simulink model "model_new"  (R2016b)
settings: Solver=FixedStepAuto  StartTime=0.0  StopTime=10.0  RelTol=1e-3
undefined symbols (not defined in the file): magnitude
settings Model: Creator=202008840  LastModifiedBy=202008840
settings OptimizationCC: DefaultParameterBehavior=Inlined  UseDivisionForNetSlopeComputation=on  UseFloatMulNetSlope=on  InlineInvariantSignals=on  PassReuseOutputArgsAs=Individual arguments  ZeroExternalMemoryAtStartup=off  ZeroInternalMemoryAtStartup=off  NoFixptDivByZeroProtection=on  EfficientFloat2IntCast=on  LifeSpan=1
settings DebuggingCC: ParameterTunabilityLossMsg=error
settings RTWCC: SystemTargetFile=ert.tlc  TemplateMakefile=ert_default_tmf  Description=Embedded Coder  GenerateReport=on  IncludeHyperlinkInReport=on  LaunchReport=on  GenerateTraceInfo=on  GenerateTraceReport=on  GenerateTraceReportSl=on  GenerateTraceReportSf=on  GenerateTraceReportEml=on  GenerateCodeMetricsReport=on
settings CodeAppCC: ForceParamTrailComments=on  IgnoreCustomStorageClasses=off  OperatorAnnotations=on  SimulinkDataObjDesc=on  SFDataObjDesc=on  MATLABFcnDesc=on  CustomSymbolStrGlobalVar=rt$N$M  CustomSymbolStrType=$N$M  CustomSymbolStrFcn=$N$M$F  CustomSymbolStrMacro=$N$M  InsertBlockDesc=on  MATLABSourceComments=on
settings ERTTargetCC: TargetLangStandard=C99 (ISO)  GenerateSampleERTMain=on  CombineSignalStateStructs=on  SupportAbsoluteTime=off  SupportComplex=off  SupportContinuousTime=on  InlinedParameterPlacement=NonHierarchical  ERTCustomFileTemplate=example_file_process.tlc  ERTFilePackagingFormat=CompactWithDataFile

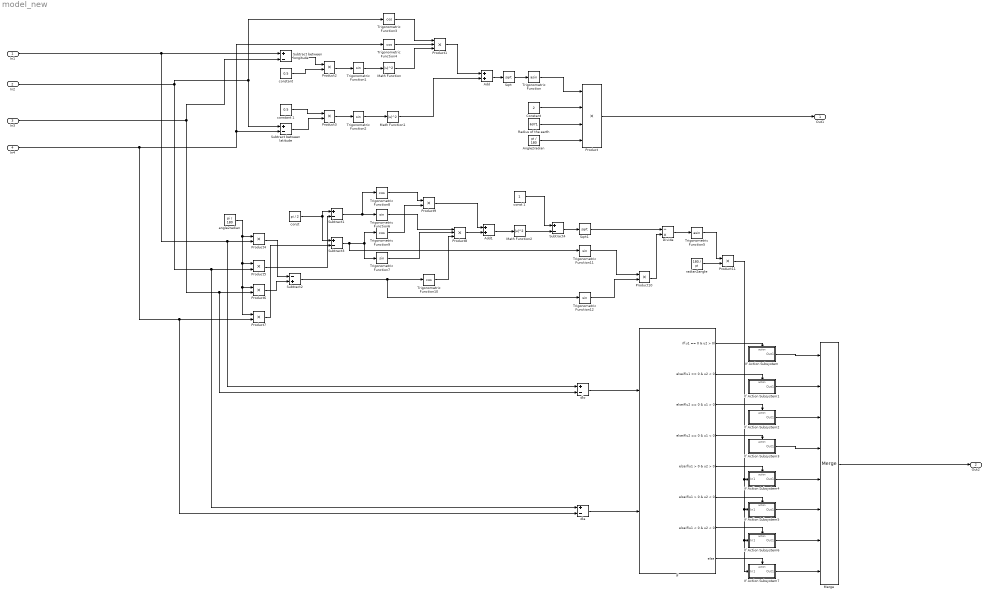
== system model_new ==
  In1 : Inport
  In2 : Inport  Port=2
  In3 : Inport  Port=3
  In4 : Inport  Port=4
  Add : Sum
  Add1 : Sum
  Angle2radian : Constant  Value=pi / 180
  Constant : Constant  Value=2
  Divide : Product  Inputs=/*
  If : If  NumInputs=2  IfExpression=u1 == 0 & u2 > 0  ElseIfExpressions=u1 == 0 & u2 < 0, u2 == 0 & u1 > 0, u2 == 0 & u1 < 0, u1 > 0 & u2 > 0, u1 > 0 & u2 < 0, u1 < 0 & u2 < 0
  If Action Subsystem : Subsystem  TreatAsAtomicUnit=on
  If Action Subsystem1 : Subsystem  TreatAsAtomicUnit=on
  If Action Subsystem2 : Subsystem  TreatAsAtomicUnit=on
  If Action Subsystem3 : Subsystem  TreatAsAtomicUnit=on
  If Action Subsystem4 : Subsystem  TreatAsAtomicUnit=on
  If Action Subsystem5 : Subsystem  TreatAsAtomicUnit=on
  If Action Subsystem6 : Subsystem  TreatAsAtomicUnit=on
  If Action Subsystem7 : Subsystem  TreatAsAtomicUnit=on
  Math Function : Math  Operator=magnitude^2  SaturateOnIntegerOverflow=on
  Math Function1 : Math  Operator=magnitude^2  SaturateOnIntegerOverflow=on
  Math Function2 : Math  Operator=magnitude^2  SaturateOnIntegerOverflow=on
  Merge : Merge  Inputs=8
  Product : Product  Inputs=4
  Product1 : Product  Inputs=3
  Product{2..7,9..11} (9 alike) : Product
  Product8 : Product  Inputs=3
  Radius of the earth : Constant  Value=6371
  Sqrt : Sqrt  SaturateOnIntegerOverflow=on
  Sqrt1 : Sqrt  SaturateOnIntegerOverflow=on
  Subtract between latitude : Sum  Inputs=+-
  Subtract between longitude : Sum  Inputs=+-
  Subtract1 : Sum  Inputs=+-
  Subtract2 : Sum  Inputs=-+
  Subtract3 : Sum  Inputs=+-
  Subtract4 : Sum  Inputs=+-
  Trigonometric Function : Trigonometry  Operator=asin
  Trigonometric Function{1..2,6..7,11..12} (6 alike) : Trigonometry
  Trigonometric Function{3..4,8..10} (5 alike) : Trigonometry  Operator=cos
  Trigonometric Function5 : Trigonometry  Operator=asin
  angle2radian : Constant  Value=pi / 180
  const : Constant  Value=pi / 2
  const 1 : Constant
  "constant " : Constant  Value=0.5
  constant 1 : Constant  Value=0.5
  dla : Sum  Inputs=+-
  dlo : Sum  Inputs=+-
  radian2angle : Constant  Value=180 / pi
  Out1 : Outport
  Out2 : Outport  Port=2
  wires:
  In4/1 -> dla/2, Product7/2, Trigonometric Function4/1, Subtract between latitude/2
  Subtract between longitude/1 -> Product2/1
  "constant "/1 -> Product2/2
  constant 1/1 -> Product3/1
  Subtract between latitude/1 -> Product3/2
  Product2/1 -> Trigonometric Function1/1
  Product3/1 -> Trigonometric Function2/1
  Trigonometric Function1/1 -> Math Function/1
  Trigonometric Function2/1 -> Math Function1/1
  Trigonometric Function3/1 -> Product1/1
  Trigonometric Function4/1 -> Product1/2
  Math Function/1 -> Product1/3
  Math Function1/1 -> Add/2
  Product1/1 -> Add/1
  Add/1 -> Sqrt/1
  Sqrt/1 -> Trigonometric Function/1
  Trigonometric Function/1 -> Product/1
  Constant/1 -> Product/2
  Radius of the earth/1 -> Product/3
  Angle2radian/1 -> Product/4
  Product/1 -> Out1/1
  In1/1 -> dlo/1, Product4/2, Subtract between longitude/1
  In2/1 -> Subtract between latitude/1, Trigonometric Function3/1, dla/1, Product5/2
  In3/1 -> dlo/2, Product6/2, Subtract between longitude/2
  angle2radian/1 -> Product7/1, Product6/1, Product5/1, Product4/1
  const/1 -> Subtract1/1, Subtract3/1
  Subtract2/1 -> Trigonometric Function12/1, Trigonometric Function10/1
  Subtract1/1 -> Trigonometric Function8/1, Trigonometric Function6/1
  Subtract3/1 -> Trigonometric Function11/1, Trigonometric Function9/1, Trigonometric Function7/1
  Trigonometric Function6/1 -> Product8/1
  Trigonometric Function7/1 -> Product8/2
  Trigonometric Function8/1 -> Product9/1
  Trigonometric Function9/1 -> Product9/2
  Trigonometric Function10/1 -> Product8/3
  Product9/1 -> Add1/1
  Product8/1 -> Add1/2
  const 1/1 -> Subtract4/1
  Subtract4/1 -> Sqrt1/1
  Add1/1 -> Math Function2/1
  Math Function2/1 -> Subtract4/2
  Trigonometric Function11/1 -> Product10/1
  Trigonometric Function12/1 -> Product10/2
  Product10/1 -> Divide/2
  Sqrt1/1 -> Divide/1
  Divide/1 -> Trigonometric Function5/1
  Trigonometric Function5/1 -> Product11/1
  radian2angle/1 -> Product11/2
  Product11/1 -> If Action Subsystem7/1(In1), If Action Subsystem6/1(In1), If Action Subsystem5/1(In1), If Action Subsystem4/1(In1)
  Product4/1 -> Subtract2/1
  Product5/1 -> Subtract1/2
  Product6/1 -> Subtract2/2
  Product7/1 -> Subtract3/2
  dlo/1 -> If/1
  dla/1 -> If/2
  If/2 -> If Action Subsystem1/Action
  If/1 -> If Action Subsystem/Action
  If/3 -> If Action Subsystem2/Action
  If/4 -> If Action Subsystem3/Action
  If/5 -> If Action Subsystem4/Action
  If/6 -> If Action Subsystem5/Action
  If/7 -> If Action Subsystem6/Action
  If/8 -> If Action Subsystem7/Action
  If Action Subsystem/1(Out1) -> Merge/1
  If Action Subsystem1/1(Out1) -> Merge/2
  If Action Subsystem2/1(Out1) -> Merge/3
  If Action Subsystem3/1(Out1) -> Merge/4
  If Action Subsystem4/1(Out1) -> Merge/5
  If Action Subsystem5/1(Out1) -> Merge/6
  If Action Subsystem6/1(Out1) -> Merge/7
  If Action Subsystem7/1(Out1) -> Merge/8
  Merge/1 -> Out2/1

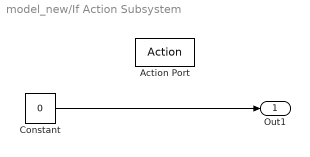
== system model_new/If Action Subsystem ==
  Action Port : ActionPort  ActionType=then
  Constant : Constant  Value=0
  Out1 : Outport
  wires:
  Constant/1 -> Out1/1

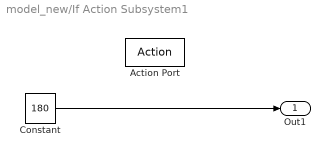
== system model_new/If Action Subsystem1 ==
  Action Port : ActionPort  ActionType=elseif
  Constant : Constant  Value=180
  Out1 : Outport
  wires:
  Constant/1 -> Out1/1

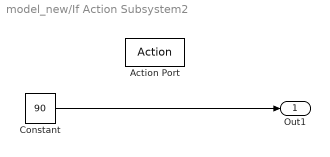
== system model_new/If Action Subsystem2 ==
  Action Port : ActionPort  ActionType=elseif
  Constant : Constant  Value=90
  Out1 : Outport
  wires:
  Constant/1 -> Out1/1

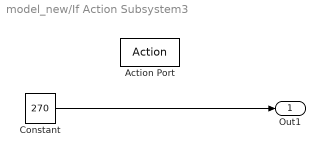
== system model_new/If Action Subsystem3 ==
  Action Port : ActionPort  ActionType=elseif
  Constant : Constant  Value=270
  Out1 : Outport
  wires:
  Constant/1 -> Out1/1

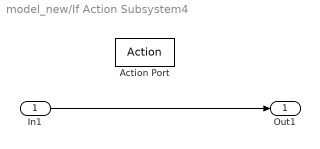
== system model_new/If Action Subsystem4 ==
  In1 : Inport
  Action Port : ActionPort  ActionType=elseif
  Out1 : Outport
  wires:
  In1/1 -> Out1/1

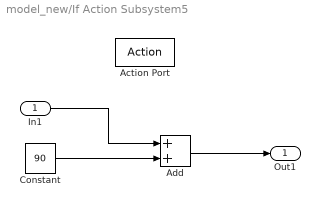
== system model_new/If Action Subsystem5 ==
  In1 : Inport
  Action Port : ActionPort  ActionType=elseif
  Add : Sum
  Constant : Constant  Value=90
  Out1 : Outport
  wires:
  Constant/1 -> Add/2
  In1/1 -> Add/1
  Add/1 -> Out1/1

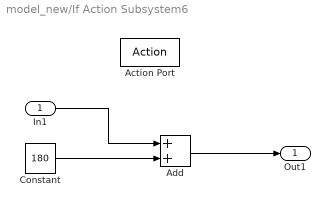
== system model_new/If Action Subsystem6 ==
  In1 : Inport
  Action Port : ActionPort  ActionType=elseif
  Add : Sum
  Constant : Constant  Value=180
  Out1 : Outport
  wires:
  Constant/1 -> Add/2
  In1/1 -> Add/1
  Add/1 -> Out1/1

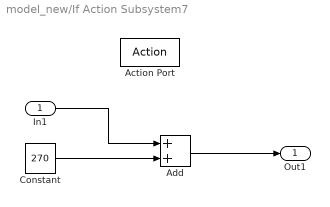
== system model_new/If Action Subsystem7 ==
  In1 : Inport
  Action Port : ActionPort  ActionType=else
  Add : Sum
  Constant : Constant  Value=270
  Out1 : Outport
  wires:
  Constant/1 -> Add/2
  In1/1 -> Add/1
  Add/1 -> Out1/1
